simulink model "EHB_speedgoat_R2020a_V1"  (R2020a)
settings: Solver=FixedStepDiscrete  StartTime=0.0  StopTime=inf  FixedStep=0.001  RelTol=1e-3  EnableMultiTasking=on
model workspace (MAT data in the model file):
  A : Simulink.Signal (value not decoded)
  B : Simulink.Signal (value not decoded)
  C : Simulink.Signal (value not decoded)
  D : Simulink.Signal (value not decoded)
  E : Simulink.Signal (value not decoded)
  calin = [-9.96 -7.98 -5.98 -3.99 -1.994 0 1.995 3.992 5.99 7.98 9.97]
  calout = [-10 -8 -6 -4 -2 0 2 4 6 8 10]
symbols that are objects in the model workspace (value not decoded): C, D
undefined symbols (not defined in the file): Com1, none, ts_IO612
libraries: simulink x1436, xpcethercatlib x1223, yisutbxlib_utilities x256, xpcutilitieslib x156, hdlsllib x145, canmsglib x46, speedgoatlib_IO602_4 x11, speedgoatlib_IO611 x7, slrttcplib x4, CanManageLib x3, slrtlib x3, xpcseriallib x2
(part 3 of 30)

== system EHB_speedgoat_R2020a_V1/PowerCtrl/PowerCtrl/CurrSet1 ==
  CurrSet[A] : Inport
  Trigger : TriggerPort  VariantControl=(inherit)  PortDimensions=1
  A2mA : Gain  Gain=1000  OutDataTypeStr=Inherit: Inherit via back propagation
  "Byte Packing " : xpcutilitieslib/Byte Packing   MaskPackedDataType=uint8  MaskUnpackedDataTypes={'uint16'}  MaskAlignment=1
  Byte Packing 1 : xpcutilitieslib/Byte Packing   MaskPackedDataType=uint8  MaskUnpackedDataTypes={'uint16'}  MaskAlignment=1
  CAN Pack : canmsglib/CAN Pack  MsgList=(none)  MsgName=CAN Msg  MsgIDType=Standard (11-bit identifier)  MsgIdentifier=1537  MsgLength=8  Remote=off  ApplyMinMax=off  BusOutput=on  SignalInfo={}
      settings: SourceProductBaseCode=ME,VN  DataFormat=raw data
  CANDataPack_ToUDP : Subsystem
  FunCode : Constant  Value=0x23  OutDataTypeStr=Inherit: Inherit via back propagation
  Index : Constant  Value=0x3003  OutDataTypeStr=Inherit: Inherit via back propagation
  Mux : Mux  Inputs=5
  SubIndex : Constant  Value=0x05  VectorParams1D=off  OutDataTypeStr=Inherit: Inherit via back propagation
  puppet : Constant  Value=[0 0]  OutDataTypeStr=Inherit: Inherit via back propagation
  Output : Outport
  wires:
  CurrSet[A]/1 -> A2mA/1
  puppet/1 -> Mux/5
  SubIndex/1 -> Mux/3
  Index/1 -> "Byte Packing "/1
  A2mA/1 -> Byte Packing 1/1
  Mux/1 -> CAN Pack/1
  "Byte Packing "/1 -> Mux/2
  CAN Pack/1 -> CANDataPack_ToUDP/1(In1)
  Byte Packing 1/1 -> Mux/4
  FunCode/1 -> Mux/1
  CANDataPack_ToUDP/1(Output) -> Output/1

== system EHB_speedgoat_R2020a_V1/PowerCtrl/PowerCtrl/Enable1 ==
  OnOff : Inport
  Trigger : TriggerPort  VariantControl=(inherit)  PortDimensions=1
  "Byte Packing " : xpcutilitieslib/Byte Packing   MaskPackedDataType=uint8  MaskUnpackedDataTypes={'uint16'}  MaskAlignment=1
  CAN Pack1 : canmsglib/CAN Pack  MsgList=(none)  MsgName=CAN Msg  MsgIDType=Standard (11-bit identifier)  MsgIdentifier=1537  MsgLength=8  Remote=off  ApplyMinMax=off  BusOutput=on  SignalInfo={}
      settings: SourceProductBaseCode=ME,VN  DataFormat=raw data
  CANDataPack_ToUDP : Subsystem
  FunCode : Constant  Value=0x2F  OutDataTypeStr=Inherit: Inherit via back propagation
  Index : Constant  Value=0x3002  OutDataTypeStr=Inherit: Inherit via back propagation
  Mux1 : Mux  Inputs=5
  SubIndex : Constant  Value=0x04  VectorParams1D=off  OutDataTypeStr=Inherit: Inherit via back propagation
  puppet : Constant  Value=[0 0 0]  OutDataTypeStr=Inherit: Inherit via back propagation
  Output : Outport
  wires:
  FunCode/1 -> Mux1/1
  puppet/1 -> Mux1/5
  SubIndex/1 -> Mux1/3
  Mux1/1 -> CAN Pack1/1
  CAN Pack1/1 -> CANDataPack_ToUDP/1(In1)
  OnOff/1 -> Mux1/4
  "Byte Packing "/1 -> Mux1/2
  Index/1 -> "Byte Packing "/1
  CANDataPack_ToUDP/1(Output) -> Output/1

== system EHB_speedgoat_R2020a_V1/PowerCtrl/PowerCtrl/IT_M3902D_Ctrl_Trigger ==
  VoltValue : Inport
  OnOff : Inport  Port=2
  CurrSet : Inport  Port=3
  PowerPosSet : Inport  Port=4
  Data Type Conversion : DataTypeConversion
  Data Type Conversion1 : DataTypeConversion
  Data Type Conversion2 : DataTypeConversion  Commented=on
  Detect Change : simulink/Logic and Bit Operations/Detect Change  vinit=0  OutDataTypeStr=boolean
  Mux : Mux  Inputs=5
  Pulse Generator : DiscretePulseGenerator  Commented=on  PulseType=Time based  Period=1  PulseWidth=50
  HVRealy_Ctrl_Trigger : Outport
  wires:
  Detect Change/1 -> HVRealy_Ctrl_Trigger/1  "HVRealy_Ctrl_Trigger"
  Mux/1 -> Detect Change/1
  CurrSet/1 -> Mux/3
  PowerPosSet/1 -> Mux/4
  VoltValue/1 -> Data Type Conversion/1
  OnOff/1 -> Data Type Conversion1/1
  Data Type Conversion/1 -> Mux/1
  Data Type Conversion1/1 -> Mux/2
  Pulse Generator/1 -> Data Type Conversion2/1
  Data Type Conversion2/1 -> Mux/5

== system EHB_speedgoat_R2020a_V1/PowerCtrl/PowerCtrl/PowerPosSet1 ==
  PowerPosSet[W] : Inport
  Trigger : TriggerPort  VariantControl=(inherit)  PortDimensions=1
  "Byte Packing " : xpcutilitieslib/Byte Packing   MaskPackedDataType=uint8  MaskUnpackedDataTypes={'uint16'}  MaskAlignment=1
  Byte Packing 1 : xpcutilitieslib/Byte Packing   MaskPackedDataType=uint8  MaskUnpackedDataTypes={'uint16'}  MaskAlignment=1
  CAN Pack : canmsglib/CAN Pack  MsgList=(none)  MsgName=CAN Msg  MsgIDType=Standard (11-bit identifier)  MsgIdentifier=1537  MsgLength=8  Remote=off  ApplyMinMax=off  BusOutput=on  SignalInfo={}
      settings: SourceProductBaseCode=ME,VN  DataFormat=raw data
  CANDataPack_ToUDP : Subsystem
  FunCode : Constant  Value=0x23  OutDataTypeStr=Inherit: Inherit via back propagation
  Index : Constant  Value=0x3003  OutDataTypeStr=Inherit: Inherit via back propagation
  Mux : Mux  Inputs=5
  SubIndex : Constant  Value=0x0E  VectorParams1D=off  OutDataTypeStr=Inherit: Inherit via back propagation
  W2mW : Gain  Gain=1000  OutDataTypeStr=Inherit: Inherit via back propagation
  puppet : Constant  Value=[0 0]  OutDataTypeStr=Inherit: Inherit via back propagation
  Output : Outport
  wires:
  PowerPosSet[W]/1 -> W2mW/1
  puppet/1 -> Mux/5
  SubIndex/1 -> Mux/3
  Index/1 -> "Byte Packing "/1
  Mux/1 -> CAN Pack/1
  "Byte Packing "/1 -> Mux/2
  CAN Pack/1 -> CANDataPack_ToUDP/1(In1)
  W2mW/1 -> Byte Packing 1/1
  FunCode/1 -> Mux/1
  Byte Packing 1/1 -> Mux/4
  CANDataPack_ToUDP/1(Output) -> Output/1

== system EHB_speedgoat_R2020a_V1/PowerCtrl/PowerCtrl/VoltSet1 ==
  VoltValue[V] : Inport
  Trigger : TriggerPort  VariantControl=(inherit)  PortDimensions=1
  "Byte Packing " : xpcutilitieslib/Byte Packing   MaskPackedDataType=uint8  MaskUnpackedDataTypes={'uint16'}  MaskAlignment=1
  Byte Packing 1 : xpcutilitieslib/Byte Packing   MaskPackedDataType=uint8  MaskUnpackedDataTypes={'uint32'}  MaskAlignment=1
  CAN Pack : canmsglib/CAN Pack  MsgList=(none)  MsgName=CAN Msg  MsgIDType=Standard (11-bit identifier)  MsgIdentifier=1537  MsgLength=8  Remote=off  ApplyMinMax=off  BusOutput=on  SignalInfo={}
      settings: SourceProductBaseCode=ME,VN  DataFormat=raw data
  CANDataPack_ToUDP : Subsystem
  FunCode : Constant  Value=0x23  OutDataTypeStr=Inherit: Inherit via back propagation
  Index : Constant  Value=0x3003  OutDataTypeStr=Inherit: Inherit via back propagation
  Mux : Mux
  SubIndex : Constant  Value=0x02  VectorParams1D=off  OutDataTypeStr=Inherit: Inherit via back propagation
  V2mV : Gain  Gain=1000  OutDataTypeStr=Inherit: Inherit via back propagation
  Output : Outport
  wires:
  FunCode/1 -> Mux/1
  Byte Packing 1/1 -> Mux/4
  CAN Pack/1 -> CANDataPack_ToUDP/1(In1)
  "Byte Packing "/1 -> Mux/2
  Mux/1 -> CAN Pack/1
  V2mV/1 -> Byte Packing 1/1
  Index/1 -> "Byte Packing "/1
  SubIndex/1 -> Mux/3
  VoltValue[V]/1 -> V2mV/1
  CANDataPack_ToUDP/1(Output) -> Output/1

== system EHB_speedgoat_R2020a_V1/TIF_04/CB2020_1/ADC ==
  DTCB CH1 : DataTypeConversion  OutDataTypeStr=double
  DTCB CH2 : DataTypeConversion  OutDataTypeStr=double
  DTCB CH3 : DataTypeConversion  OutDataTypeStr=double
  EtherCAT PDO Receive ADC CH1 : xpcethercatlib/EtherCAT PDO Receive  Priority=2  sig_name=Box 5 (CB2020).PDOGetValue process data mapping.adcvalue1  sig_offset=10808  sig_type=uint16  type_size=16  sig_dim=1  device_id=0  sample_time=0.001000
      settings: SourceProductBaseCode=XP
  EtherCAT PDO Receive ADC CH2 : xpcethercatlib/EtherCAT PDO Receive  Priority=2  sig_name=Box 5 (CB2020).PDOGetValue process data mapping.adcvalue2  sig_offset=10824  sig_type=uint16  type_size=16  sig_dim=1  device_id=0  sample_time=0.001000
      settings: SourceProductBaseCode=XP
  EtherCAT PDO Receive ADC CH3 : xpcethercatlib/EtherCAT PDO Receive  Priority=2  sig_name=Box 5 (CB2020).PDOGetValue process data mapping.adcvalue3  sig_offset=10840  sig_type=uint16  type_size=16  sig_dim=1  device_id=0  sample_time=0.001000
      settings: SourceProductBaseCode=XP
  Gain CH1 : Gain  Gain=1/1000
  Gain CH2 : Gain  Gain=1/1000
  Gain CH3 : Gain  Gain=1/1000
  ADC_CH1[V] : Outport
  ADC_CH2[V] : Outport  Port=2
  ADC_CH3[V] : Outport  Port=3
  wires:
  EtherCAT PDO Receive ADC CH1/1 -> DTCB CH1/1
  DTCB CH1/1 -> Gain CH1/1
  Gain CH1/1 -> ADC_CH1[V]/1  "ADC_CH1[V]"
  EtherCAT PDO Receive ADC CH2/1 -> DTCB CH2/1
  DTCB CH2/1 -> Gain CH2/1
  Gain CH2/1 -> ADC_CH2[V]/1  "ADC_CH2[V]"
  EtherCAT PDO Receive ADC CH3/1 -> DTCB CH3/1
  DTCB CH3/1 -> Gain CH3/1
  Gain CH3/1 -> ADC_CH3[V]/1  "ADC_CH3[V]"

== system EHB_speedgoat_R2020a_V1/TIF_04/CB2020_1/AI1 ==
  Vol : Inport
  Add : Sum  Inputs=-+
  Constant : Constant  Value=4.9874
  V2A : Gain  Gain=1/0.1  OutDataTypeStr=Inherit: Inherit via back propagation
  Cur : Outport
  wires:
  Add/1 -> V2A/1
  Vol/1 -> Add/2
  Constant/1 -> Add/1
  V2A/1 -> Cur/1

== system EHB_speedgoat_R2020a_V1/TIF_04/CB2020_1/AI2 ==
  Vol : Inport
  Add : Sum  Inputs=-+
  Constant : Constant  Value=5.0067
  V2A : Gain  Gain=1/0.1  OutDataTypeStr=Inherit: Inherit via back propagation
  Cur : Outport
  wires:
  V2A/1 -> Cur/1
  Constant/1 -> Add/1
  Vol/1 -> Add/2
  Add/1 -> V2A/1

== system EHB_speedgoat_R2020a_V1/TIF_04/CB2020_1/AI3 ==
  Vol : Inport
  Add : Sum  Inputs=-+
  Constant : Constant  Value=4.9975
  V2A : Gain  Gain=1/0.1  OutDataTypeStr=Inherit: Inherit via back propagation
  Cur : Outport
  wires:
  Add/1 -> V2A/1
  Vol/1 -> Add/2
  Constant/1 -> Add/1
  V2A/1 -> Cur/1

== system EHB_speedgoat_R2020a_V1/TIF_04/CB2020_1/DAC1 ==
  DAC_CH1[V] : Inport
  DAC_CH1_CAL[V] : Constant  Value=0
  EtherCAT PDO Transmit DAC CH1 : xpcethercatlib/EtherCAT PDO Transmit   Priority=3  sig_name=Box 5 (CB2020).PDOSetValue process data mapping.dacvalue1  sig_offset=10808  sig_type=int16  type_size=16  sig_dim=1  device_id=0  sample_time=0.001000
      settings: SourceProductBaseCode=XP
  dp2c CH1 : Subsystem  mask(dacphy2cmd){}
  wires:
  DAC_CH1[V]/1 -> dp2c CH1/1(dac_value)
  DAC_CH1_CAL[V]/1 -> dp2c CH1/2(dac_value_calibrate)
  dp2c CH1/1(cmd_value) -> EtherCAT PDO Transmit DAC CH1/1

== system EHB_speedgoat_R2020a_V1/TIF_04/CB2020_1/mean1 ==
  In1 : Inport
  Add : Sum  Inputs=++++
  Add{1..4} (4 alike) : Sum  Inputs=++++++++++++++++++++
  Delay{,1..79} (80 alike) : Delay  DelayLength=1
  Gain : Gain  Gain=1/80
  Vol : Outport
  wires:
  Add/1 -> Gain/1
  Gain/1 -> Vol/1
  Delay36/1 -> Delay37/1, Add2/7
  Delay37/1 -> Delay38/1, Add2/8
  Delay34/1 -> Delay35/1, Add2/5
  Delay33/1 -> Delay34/1, Add2/4
  Delay20/1 -> Delay21/1, Add2/1
  Delay32/1 -> Delay33/1, Add2/3
  Add2/1 -> Add/2
  Delay35/1 -> Delay36/1, Add2/6
  Delay21/1 -> Delay32/1, Add2/2
  Delay38/1 -> Delay39/1, Add2/9
  Delay39/1 -> Delay22/1, Add2/10
  Delay19/1 -> Add1/20, Delay20/1
  Delay30/1 -> Delay31/1, Add2/19
  Delay23/1 -> Delay24/1, Add2/12
  Delay27/1 -> Delay28/1, Add2/16
  Delay24/1 -> Delay25/1, Add2/13
  Delay22/1 -> Delay23/1, Add2/11
  Delay25/1 -> Delay26/1, Add2/14
  Delay26/1 -> Delay27/1, Add2/15
  Delay29/1 -> Delay30/1, Add2/18
  Delay28/1 -> Delay29/1, Add2/17
  Delay16/1 -> Add1/17, Delay17/1
  Delay17/1 -> Add1/18, Delay18/1
  Delay14/1 -> Add1/15, Delay15/1
  Delay13/1 -> Add1/14, Delay14/1
  Delay10/1 -> Add1/11, Delay11/1
  Delay12/1 -> Add1/13, Delay13/1
  Delay15/1 -> Add1/16, Delay16/1
  Delay11/1 -> Add1/12, Delay12/1
  Delay18/1 -> Add1/19, Delay19/1
  In1/1 -> Delay/1
  Delay9/1 -> Add1/10, Delay10/1
  Delay8/1 -> Add1/9, Delay9/1
  Delay1/1 -> Add1/2, Delay2/1
  Delay5/1 -> Add1/6, Delay6/1
  Add1/1 -> Add/1
  Delay2/1 -> Add1/3, Delay3/1
  Delay/1 -> Add1/1, Delay1/1
  Delay3/1 -> Add1/4, Delay4/1
  Delay4/1 -> Add1/5, Delay5/1
  Delay7/1 -> Add1/8, Delay8/1
  Delay6/1 -> Add1/7, Delay7/1
  Delay48/1 -> Add3/17, Delay49/1
  Delay49/1 -> Add3/18, Delay50/1
  Delay46/1 -> Add3/15, Delay47/1
  Delay45/1 -> Add3/14, Delay46/1
  Delay42/1 -> Add3/11, Delay43/1
  Delay44/1 -> Add3/13, Delay45/1
  Delay47/1 -> Add3/16, Delay48/1
  Delay43/1 -> Add3/12, Delay44/1
  Delay50/1 -> Add3/19, Delay51/1
  Delay31/1 -> Delay40/1, Add2/20
  Delay59/1 -> Add3/10, Delay42/1
  Delay58/1 -> Add3/9, Delay59/1
  Delay41/1 -> Add3/2, Delay52/1
  Delay55/1 -> Add3/6, Delay56/1
  Add3/1 -> Add/3
  Delay52/1 -> Add3/3, Delay53/1
  Delay40/1 -> Add3/1, Delay41/1
  Delay53/1 -> Add3/4, Delay54/1
  Delay54/1 -> Add3/5, Delay55/1
  Delay57/1 -> Add3/8, Delay58/1
  Delay56/1 -> Add3/7, Delay57/1
  Delay76/1 -> Delay77/1, Add4/7
  Delay77/1 -> Delay78/1, Add4/8
  Delay74/1 -> Delay75/1, Add4/5
  Delay73/1 -> Delay74/1, Add4/4
  Delay60/1 -> Delay61/1, Add4/1
  Delay72/1 -> Delay73/1, Add4/3
  Add4/1 -> Add/4
  Delay75/1 -> Delay76/1, Add4/6
  Delay61/1 -> Delay72/1, Add4/2
  Delay78/1 -> Delay79/1, Add4/9
  Delay79/1 -> Delay62/1, Add4/10
  Delay71/1 -> Add4/20
  Delay51/1 -> Delay60/1, Add3/20
  Delay70/1 -> Delay71/1, Add4/19
  Delay63/1 -> Delay64/1, Add4/12
  Delay67/1 -> Delay68/1, Add4/16
  Delay64/1 -> Delay65/1, Add4/13
  Delay62/1 -> Delay63/1, Add4/11
  Delay65/1 -> Delay66/1, Add4/14
  Delay66/1 -> Delay67/1, Add4/15
  Delay69/1 -> Delay70/1, Add4/18
  Delay68/1 -> Delay69/1, Add4/17

== system EHB_speedgoat_R2020a_V1/TIF_04/CB2020_1/mean2 ==
  In1 : Inport
  Add : Sum  Inputs=++++
  Add{1..4} (4 alike) : Sum  Inputs=++++++++++++++++++++
  Delay{,1..79} (80 alike) : Delay  DelayLength=1
  Gain : Gain  Gain=1/80
  Vol : Outport
  wires:
  Delay68/1 -> Add4/17, Delay69/1
  Delay69/1 -> Add4/18, Delay70/1
  Delay66/1 -> Add4/15, Delay67/1
  Delay65/1 -> Add4/14, Delay66/1
  Delay62/1 -> Add4/11, Delay63/1
  Delay64/1 -> Add4/13, Delay65/1
  Delay67/1 -> Add4/16, Delay68/1
  Delay63/1 -> Add4/12, Delay64/1
  Delay70/1 -> Add4/19, Delay71/1
  Delay51/1 -> Add3/20, Delay60/1
  Delay71/1 -> Add4/20
  Delay79/1 -> Add4/10, Delay62/1
  Delay78/1 -> Add4/9, Delay79/1
  Delay61/1 -> Add4/2, Delay72/1
  Delay75/1 -> Add4/6, Delay76/1
  Add4/1 -> Add/4
  Delay72/1 -> Add4/3, Delay73/1
  Delay60/1 -> Add4/1, Delay61/1
  Delay73/1 -> Add4/4, Delay74/1
  Delay74/1 -> Add4/5, Delay75/1
  Delay77/1 -> Add4/8, Delay78/1
  Delay76/1 -> Add4/7, Delay77/1
  Delay56/1 -> Delay57/1, Add3/7
  Delay57/1 -> Delay58/1, Add3/8
  Delay54/1 -> Delay55/1, Add3/5
  Delay53/1 -> Delay54/1, Add3/4
  Delay40/1 -> Delay41/1, Add3/1
  Delay52/1 -> Delay53/1, Add3/3
  Add3/1 -> Add/3
  Delay55/1 -> Delay56/1, Add3/6
  Delay41/1 -> Delay52/1, Add3/2
  Delay58/1 -> Delay59/1, Add3/9
  Delay59/1 -> Delay42/1, Add3/10
  Delay31/1 -> Add2/20, Delay40/1
  Delay50/1 -> Delay51/1, Add3/19
  Delay43/1 -> Delay44/1, Add3/12
  Delay47/1 -> Delay48/1, Add3/16
  Delay44/1 -> Delay45/1, Add3/13
  Delay42/1 -> Delay43/1, Add3/11
  Delay45/1 -> Delay46/1, Add3/14
  Delay46/1 -> Delay47/1, Add3/15
  Delay49/1 -> Delay50/1, Add3/18
  Delay48/1 -> Delay49/1, Add3/17
  Delay6/1 -> Delay7/1, Add1/7
  Delay7/1 -> Delay8/1, Add1/8
  Delay4/1 -> Delay5/1, Add1/5
  Delay3/1 -> Delay4/1, Add1/4
  Delay/1 -> Delay1/1, Add1/1
  Delay2/1 -> Delay3/1, Add1/3
  Add1/1 -> Add/1
  Delay5/1 -> Delay6/1, Add1/6
  Delay1/1 -> Delay2/1, Add1/2
  Delay8/1 -> Delay9/1, Add1/9
  Delay9/1 -> Delay10/1, Add1/10
  In1/1 -> Delay/1
  Delay18/1 -> Delay19/1, Add1/19
  Delay11/1 -> Delay12/1, Add1/12
  Delay15/1 -> Delay16/1, Add1/16
  Delay12/1 -> Delay13/1, Add1/13
  Delay10/1 -> Delay11/1, Add1/11
  Delay13/1 -> Delay14/1, Add1/14
  Delay14/1 -> Delay15/1, Add1/15
  Delay17/1 -> Delay18/1, Add1/18
  Delay16/1 -> Delay17/1, Add1/17
  Delay28/1 -> Add2/17, Delay29/1
  Delay29/1 -> Add2/18, Delay30/1
  Delay26/1 -> Add2/15, Delay27/1
  Delay25/1 -> Add2/14, Delay26/1
  Delay22/1 -> Add2/11, Delay23/1
  Delay24/1 -> Add2/13, Delay25/1
  Delay27/1 -> Add2/16, Delay28/1
  Delay23/1 -> Add2/12, Delay24/1
  Delay30/1 -> Add2/19, Delay31/1
  Delay19/1 -> Delay20/1, Add1/20
  Delay39/1 -> Add2/10, Delay22/1
  Delay38/1 -> Add2/9, Delay39/1
  Delay21/1 -> Add2/2, Delay32/1
  Delay35/1 -> Add2/6, Delay36/1
  Add2/1 -> Add/2
  Delay32/1 -> Add2/3, Delay33/1
  Delay20/1 -> Add2/1, Delay21/1
  Delay33/1 -> Add2/4, Delay34/1
  Delay34/1 -> Add2/5, Delay35/1
  Delay37/1 -> Add2/8, Delay38/1
  Delay36/1 -> Add2/7, Delay37/1
  Gain/1 -> Vol/1
  Add/1 -> Gain/1

== system EHB_speedgoat_R2020a_V1/TIF_04/CB2020_1/mean3 ==
  In1 : Inport
  Add : Sum  Inputs=++++
  Add{1..4} (4 alike) : Sum  Inputs=++++++++++++++++++++
  Delay{,1..79} (80 alike) : Delay  DelayLength=1
  Gain : Gain  Gain=1/80
  Vol : Outport
  wires:
  Add/1 -> Gain/1
  Gain/1 -> Vol/1
  Delay36/1 -> Delay37/1, Add2/7
  Delay37/1 -> Delay38/1, Add2/8
  Delay34/1 -> Delay35/1, Add2/5
  Delay33/1 -> Delay34/1, Add2/4
  Delay20/1 -> Delay21/1, Add2/1
  Delay32/1 -> Delay33/1, Add2/3
  Add2/1 -> Add/2
  Delay35/1 -> Delay36/1, Add2/6
  Delay21/1 -> Delay32/1, Add2/2
  Delay38/1 -> Delay39/1, Add2/9
  Delay39/1 -> Delay22/1, Add2/10
  Delay19/1 -> Add1/20, Delay20/1
  Delay30/1 -> Delay31/1, Add2/19
  Delay23/1 -> Delay24/1, Add2/12
  Delay27/1 -> Delay28/1, Add2/16
  Delay24/1 -> Delay25/1, Add2/13
  Delay22/1 -> Delay23/1, Add2/11
  Delay25/1 -> Delay26/1, Add2/14
  Delay26/1 -> Delay27/1, Add2/15
  Delay29/1 -> Delay30/1, Add2/18
  Delay28/1 -> Delay29/1, Add2/17
  Delay16/1 -> Add1/17, Delay17/1
  Delay17/1 -> Add1/18, Delay18/1
  Delay14/1 -> Add1/15, Delay15/1
  Delay13/1 -> Add1/14, Delay14/1
  Delay10/1 -> Add1/11, Delay11/1
  Delay12/1 -> Add1/13, Delay13/1
  Delay15/1 -> Add1/16, Delay16/1
  Delay11/1 -> Add1/12, Delay12/1
  Delay18/1 -> Add1/19, Delay19/1
  In1/1 -> Delay/1
  Delay9/1 -> Add1/10, Delay10/1
  Delay8/1 -> Add1/9, Delay9/1
  Delay1/1 -> Add1/2, Delay2/1
  Delay5/1 -> Add1/6, Delay6/1
  Add1/1 -> Add/1
  Delay2/1 -> Add1/3, Delay3/1
  Delay/1 -> Add1/1, Delay1/1
  Delay3/1 -> Add1/4, Delay4/1
  Delay4/1 -> Add1/5, Delay5/1
  Delay7/1 -> Add1/8, Delay8/1
  Delay6/1 -> Add1/7, Delay7/1
  Delay48/1 -> Add3/17, Delay49/1
  Delay49/1 -> Add3/18, Delay50/1
  Delay46/1 -> Add3/15, Delay47/1
  Delay45/1 -> Add3/14, Delay46/1
  Delay42/1 -> Add3/11, Delay43/1
  Delay44/1 -> Add3/13, Delay45/1
  Delay47/1 -> Add3/16, Delay48/1
  Delay43/1 -> Add3/12, Delay44/1
  Delay50/1 -> Add3/19, Delay51/1
  Delay31/1 -> Delay40/1, Add2/20
  Delay59/1 -> Add3/10, Delay42/1
  Delay58/1 -> Add3/9, Delay59/1
  Delay41/1 -> Add3/2, Delay52/1
  Delay55/1 -> Add3/6, Delay56/1
  Add3/1 -> Add/3
  Delay52/1 -> Add3/3, Delay53/1
  Delay40/1 -> Add3/1, Delay41/1
  Delay53/1 -> Add3/4, Delay54/1
  Delay54/1 -> Add3/5, Delay55/1
  Delay57/1 -> Add3/8, Delay58/1
  Delay56/1 -> Add3/7, Delay57/1
  Delay76/1 -> Delay77/1, Add4/7
  Delay77/1 -> Delay78/1, Add4/8
  Delay74/1 -> Delay75/1, Add4/5
  Delay73/1 -> Delay74/1, Add4/4
  Delay60/1 -> Delay61/1, Add4/1
  Delay72/1 -> Delay73/1, Add4/3
  Add4/1 -> Add/4
  Delay75/1 -> Delay76/1, Add4/6
  Delay61/1 -> Delay72/1, Add4/2
  Delay78/1 -> Delay79/1, Add4/9
  Delay79/1 -> Delay62/1, Add4/10
  Delay71/1 -> Add4/20
  Delay51/1 -> Delay60/1, Add3/20
  Delay70/1 -> Delay71/1, Add4/19
  Delay63/1 -> Delay64/1, Add4/12
  Delay67/1 -> Delay68/1, Add4/16
  Delay64/1 -> Delay65/1, Add4/13
  Delay62/1 -> Delay63/1, Add4/11
  Delay65/1 -> Delay66/1, Add4/14
  Delay66/1 -> Delay67/1, Add4/15
  Delay69/1 -> Delay70/1, Add4/18
  Delay68/1 -> Delay69/1, Add4/17

== system EHB_speedgoat_R2020a_V1/TIF_04/CB2020_2/ADC ==
  DTCB CH{1..16} (16 alike) : DataTypeConversion  OutDataTypeStr=double
  EtherCAT PDO Receive ADC CH1 : xpcethercatlib/EtherCAT PDO Receive  Priority=2  sig_name=Box 6 (CB2020).PDOGetValue process data mapping.adcvalue1  sig_offset=11128  sig_type=uint16  type_size=16  sig_dim=1  device_id=0  sample_time=0.001000
      settings: SourceProductBaseCode=XP
  EtherCAT PDO Receive ADC CH10 : xpcethercatlib/EtherCAT PDO Receive  Priority=2  sig_name=Box 6 (CB2020).PDOGetValue process data mapping.adcvalue10  sig_offset=11272  sig_type=uint16  type_size=16  sig_dim=1  device_id=0  sample_time=0.001000
      settings: SourceProductBaseCode=XP
  EtherCAT PDO Receive ADC CH11 : xpcethercatlib/EtherCAT PDO Receive  Priority=2  sig_name=Box 6 (CB2020).PDOGetValue process data mapping.adcvalue11  sig_offset=11288  sig_type=uint16  type_size=16  sig_dim=1  device_id=0  sample_time=0.001000
      settings: SourceProductBaseCode=XP
  EtherCAT PDO Receive ADC CH12 : xpcethercatlib/EtherCAT PDO Receive  Priority=2  sig_name=Box 6 (CB2020).PDOGetValue process data mapping.adcvalue12  sig_offset=11304  sig_type=uint16  type_size=16  sig_dim=1  device_id=0  sample_time=0.001000
      settings: SourceProductBaseCode=XP
  EtherCAT PDO Receive ADC CH13 : xpcethercatlib/EtherCAT PDO Receive  Priority=2  sig_name=Box 6 (CB2020).PDOGetValue process data mapping.adcvalue13  sig_offset=11320  sig_type=uint16  type_size=16  sig_dim=1  device_id=0  sample_time=0.001000
      settings: SourceProductBaseCode=XP
  EtherCAT PDO Receive ADC CH14 : xpcethercatlib/EtherCAT PDO Receive  Priority=2  sig_name=Box 6 (CB2020).PDOGetValue process data mapping.adcvalue14  sig_offset=11336  sig_type=uint16  type_size=16  sig_dim=1  device_id=0  sample_time=0.001000
      settings: SourceProductBaseCode=XP
  EtherCAT PDO Receive ADC CH15 : xpcethercatlib/EtherCAT PDO Receive  Priority=2  sig_name=Box 6 (CB2020).PDOGetValue process data mapping.adcvalue15  sig_offset=11352  sig_type=uint16  type_size=16  sig_dim=1  device_id=0  sample_time=0.001000
      settings: SourceProductBaseCode=XP
  EtherCAT PDO Receive ADC CH16 : xpcethercatlib/EtherCAT PDO Receive  Priority=2  sig_name=Box 6 (CB2020).PDOGetValue process data mapping.adcvalue16  sig_offset=11368  sig_type=uint16  type_size=16  sig_dim=1  device_id=0  sample_time=0.001000
      settings: SourceProductBaseCode=XP
  EtherCAT PDO Receive ADC CH2 : xpcethercatlib/EtherCAT PDO Receive  Priority=2  sig_name=Box 6 (CB2020).PDOGetValue process data mapping.adcvalue2  sig_offset=11144  sig_type=uint16  type_size=16  sig_dim=1  device_id=0  sample_time=0.001000
      settings: SourceProductBaseCode=XP
  EtherCAT PDO Receive ADC CH3 : xpcethercatlib/EtherCAT PDO Receive  Priority=2  sig_name=Box 6 (CB2020).PDOGetValue process data mapping.adcvalue3  sig_offset=11160  sig_type=uint16  type_size=16  sig_dim=1  device_id=0  sample_time=0.001000
      settings: SourceProductBaseCode=XP
  EtherCAT PDO Receive ADC CH4 : xpcethercatlib/EtherCAT PDO Receive  Priority=2  sig_name=Box 6 (CB2020).PDOGetValue process data mapping.adcvalue4  sig_offset=11176  sig_type=uint16  type_size=16  sig_dim=1  device_id=0  sample_time=0.001000
      settings: SourceProductBaseCode=XP
  EtherCAT PDO Receive ADC CH5 : xpcethercatlib/EtherCAT PDO Receive  Priority=2  sig_name=Box 6 (CB2020).PDOGetValue process data mapping.adcvalue5  sig_offset=11192  sig_type=uint16  type_size=16  sig_dim=1  device_id=0  sample_time=0.001000
      settings: SourceProductBaseCode=XP
  EtherCAT PDO Receive ADC CH6 : xpcethercatlib/EtherCAT PDO Receive  Priority=2  sig_name=Box 6 (CB2020).PDOGetValue process data mapping.adcvalue6  sig_offset=11208  sig_type=uint16  type_size=16  sig_dim=1  device_id=0  sample_time=0.001000
      settings: SourceProductBaseCode=XP
  EtherCAT PDO Receive ADC CH7 : xpcethercatlib/EtherCAT PDO Receive  Priority=2  sig_name=Box 6 (CB2020).PDOGetValue process data mapping.adcvalue7  sig_offset=11224  sig_type=uint16  type_size=16  sig_dim=1  device_id=0  sample_time=0.001000
      settings: SourceProductBaseCode=XP
  EtherCAT PDO Receive ADC CH8 : xpcethercatlib/EtherCAT PDO Receive  Priority=2  sig_name=Box 6 (CB2020).PDOGetValue process data mapping.adcvalue8  sig_offset=11240  sig_type=uint16  type_size=16  sig_dim=1  device_id=0  sample_time=0.001000
      settings: SourceProductBaseCode=XP
  EtherCAT PDO Receive ADC CH9 : xpcethercatlib/EtherCAT PDO Receive  Priority=2  sig_name=Box 6 (CB2020).PDOGetValue process data mapping.adcvalue9  sig_offset=11256  sig_type=uint16  type_size=16  sig_dim=1  device_id=0  sample_time=0.001000
      settings: SourceProductBaseCode=XP
  Gain CH{1..16} (16 alike) : Gain  Gain=1/1000
  ADC_CH1[V] : Outport
  ADC_CH2[V] : Outport  Port=2
  ADC_CH3[V] : Outport  Port=3
  ADC_CH4[V] : Outport  Port=4
  ADC_CH5[V] : Outport  Port=5
  ADC_CH6[V] : Outport  Port=6
  ADC_CH7[V] : Outport  Port=7
  ADC_CH8[V] : Outport  Port=8
  ADC_CH9[V] : Outport  Port=9
  ADC_CH10[V] : Outport  Port=10
  ADC_CH11[V] : Outport  Port=11
  ADC_CH12[V] : Outport  Port=12
  ADC_CH13[V] : Outport  Port=13
  ADC_CH14[V] : Outport  Port=14
  ADC_CH15[V] : Outport  Port=15
  ADC_CH16[V] : Outport  Port=16
  wires:
  EtherCAT PDO Receive ADC CH1/1 -> DTCB CH1/1
  DTCB CH1/1 -> Gain CH1/1
  Gain CH1/1 -> ADC_CH1[V]/1  "ADC_CH1[V]"
  EtherCAT PDO Receive ADC CH2/1 -> DTCB CH2/1
  DTCB CH2/1 -> Gain CH2/1
  Gain CH2/1 -> ADC_CH2[V]/1  "ADC_CH2[V]"
  EtherCAT PDO Receive ADC CH3/1 -> DTCB CH3/1
  DTCB CH3/1 -> Gain CH3/1
  Gain CH3/1 -> ADC_CH3[V]/1  "ADC_CH3[V]"
  EtherCAT PDO Receive ADC CH4/1 -> DTCB CH4/1
  DTCB CH4/1 -> Gain CH4/1
  Gain CH4/1 -> ADC_CH4[V]/1  "ADC_CH4[V]"
  EtherCAT PDO Receive ADC CH5/1 -> DTCB CH5/1
  DTCB CH5/1 -> Gain CH5/1
  Gain CH5/1 -> ADC_CH5[V]/1  "ADC_CH5[V]"
  EtherCAT PDO Receive ADC CH6/1 -> DTCB CH6/1
  DTCB CH6/1 -> Gain CH6/1
  Gain CH6/1 -> ADC_CH6[V]/1  "ADC_CH6[V]"
  EtherCAT PDO Receive ADC CH7/1 -> DTCB CH7/1
  DTCB CH7/1 -> Gain CH7/1
  Gain CH7/1 -> ADC_CH7[V]/1  "ADC_CH7[V]"
  EtherCAT PDO Receive ADC CH8/1 -> DTCB CH8/1
  DTCB CH8/1 -> Gain CH8/1
  Gain CH8/1 -> ADC_CH8[V]/1  "ADC_CH8[V]"
  EtherCAT PDO Receive ADC CH9/1 -> DTCB CH9/1
  DTCB CH9/1 -> Gain CH9/1
  Gain CH9/1 -> ADC_CH9[V]/1  "ADC_CH9[V]"
  EtherCAT PDO Receive ADC CH10/1 -> DTCB CH10/1
  DTCB CH10/1 -> Gain CH10/1
  Gain CH10/1 -> ADC_CH10[V]/1  "ADC_CH10[V]"
  EtherCAT PDO Receive ADC CH11/1 -> DTCB CH11/1
  DTCB CH11/1 -> Gain CH11/1
  Gain CH11/1 -> ADC_CH11[V]/1  "ADC_CH11[V]"
  EtherCAT PDO Receive ADC CH12/1 -> DTCB CH12/1
  DTCB CH12/1 -> Gain CH12/1
  Gain CH12/1 -> ADC_CH12[V]/1  "ADC_CH12[V]"
  EtherCAT PDO Receive ADC CH13/1 -> DTCB CH13/1
  DTCB CH13/1 -> Gain CH13/1
  Gain CH13/1 -> ADC_CH13[V]/1  "ADC_CH13[V]"
  EtherCAT PDO Receive ADC CH14/1 -> DTCB CH14/1
  DTCB CH14/1 -> Gain CH14/1
  Gain CH14/1 -> ADC_CH14[V]/1  "ADC_CH14[V]"
  EtherCAT PDO Receive ADC CH15/1 -> DTCB CH15/1
  DTCB CH15/1 -> Gain CH15/1
  Gain CH15/1 -> ADC_CH15[V]/1  "ADC_CH15[V]"
  EtherCAT PDO Receive ADC CH16/1 -> DTCB CH16/1
  DTCB CH16/1 -> Gain CH16/1
  Gain CH16/1 -> ADC_CH16[V]/1  "ADC_CH16[V]"

== system EHB_speedgoat_R2020a_V1/TIF_04/CB2020_2/AI1 ==
  Vol : Inport
  Add : Sum  Inputs=-+
  Constant : Constant  Value=4.976
  V2A : Gain  Gain=1/0.1  OutDataTypeStr=Inherit: Inherit via back propagation
  Cur : Outport
  wires:
  Add/1 -> V2A/1
  Vol/1 -> Add/2
  Constant/1 -> Add/1
  V2A/1 -> Cur/1

== system EHB_speedgoat_R2020a_V1/TIF_04/CB2020_2/AI10 ==
  Vol : Inport
  Add : Sum  Inputs=-+
  Constant : Constant  Value=4.9836
  V2A : Gain  Gain=1/0.1  OutDataTypeStr=Inherit: Inherit via back propagation
  Cur : Outport
  wires:
  Add/1 -> V2A/1
  Vol/1 -> Add/2
  Constant/1 -> Add/1
  V2A/1 -> Cur/1

== system EHB_speedgoat_R2020a_V1/TIF_04/CB2020_2/AI11 ==
  Vol : Inport
  Add : Sum  Inputs=-+
  Constant : Constant  Value=5.003
  V2A : Gain  Gain=1/0.1  OutDataTypeStr=Inherit: Inherit via back propagation
  Cur : Outport
  wires:
  V2A/1 -> Cur/1
  Constant/1 -> Add/1
  Vol/1 -> Add/2
  Add/1 -> V2A/1

== system EHB_speedgoat_R2020a_V1/TIF_04/CB2020_2/AI12 ==
  Vol : Inport
  Add : Sum  Inputs=-+
  Constant : Constant  Value=4.994
  V2A : Gain  Gain=1/0.1  OutDataTypeStr=Inherit: Inherit via back propagation
  Cur : Outport
  wires:
  Add/1 -> V2A/1
  Vol/1 -> Add/2
  Constant/1 -> Add/1
  V2A/1 -> Cur/1

== system EHB_speedgoat_R2020a_V1/TIF_04/CB2020_2/AI13 ==
  Vol : Inport
  Add : Sum  Inputs=-+
  Constant : Constant  Value=5
  V2A : Gain  Gain=1/0.1  OutDataTypeStr=Inherit: Inherit via back propagation
  Cur : Outport
  wires:
  V2A/1 -> Cur/1
  Constant/1 -> Add/1
  Vol/1 -> Add/2
  Add/1 -> V2A/1

== system EHB_speedgoat_R2020a_V1/TIF_04/CB2020_2/AI14 ==
  Vol : Inport
  Add : Sum  Inputs=-+
  Constant : Constant  Value=4.996
  V2A : Gain  Gain=1/0.1  OutDataTypeStr=Inherit: Inherit via back propagation
  Cur : Outport
  wires:
  V2A/1 -> Cur/1
  Constant/1 -> Add/1
  Vol/1 -> Add/2
  Add/1 -> V2A/1

== system EHB_speedgoat_R2020a_V1/TIF_04/CB2020_2/AI15 ==
  Vol : Inport
  Add : Sum  Inputs=-+
  Constant : Constant  Value=4.9926
  V2A : Gain  Gain=1/0.1  OutDataTypeStr=Inherit: Inherit via back propagation
  Cur : Outport
  wires:
  Add/1 -> V2A/1
  Vol/1 -> Add/2
  Constant/1 -> Add/1
  V2A/1 -> Cur/1

== system EHB_speedgoat_R2020a_V1/TIF_04/CB2020_2/AI16 ==
  Vol : Inport
  Add : Sum  Inputs=-+
  Constant : Constant  Value=4.996
  V2A : Gain  Gain=1/0.1  OutDataTypeStr=Inherit: Inherit via back propagation
  Cur : Outport
  wires:
  V2A/1 -> Cur/1
  Constant/1 -> Add/1
  Vol/1 -> Add/2
  Add/1 -> V2A/1

== system EHB_speedgoat_R2020a_V1/TIF_04/CB2020_2/AI2 ==
  Vol : Inport
  Add : Sum  Inputs=-+
  Constant : Constant  Value=4.9959
  V2A : Gain  Gain=1/0.1  OutDataTypeStr=Inherit: Inherit via back propagation
  Cur : Outport
  wires:
  V2A/1 -> Cur/1
  Constant/1 -> Add/1
  Vol/1 -> Add/2
  Add/1 -> V2A/1

== system EHB_speedgoat_R2020a_V1/TIF_04/CB2020_2/AI3 ==
  Vol : Inport
  Add : Sum  Inputs=-+
  Constant : Constant  Value=5.0018
  V2A : Gain  Gain=1/0.1  OutDataTypeStr=Inherit: Inherit via back propagation
  Cur : Outport
  wires:
  Add/1 -> V2A/1
  Vol/1 -> Add/2
  Constant/1 -> Add/1
  V2A/1 -> Cur/1

== system EHB_speedgoat_R2020a_V1/TIF_04/CB2020_2/AI4 ==
  Vol : Inport
  Add : Sum  Inputs=-+
  Constant : Constant  Value=5.0032
  V2A : Gain  Gain=1/0.1  OutDataTypeStr=Inherit: Inherit via back propagation
  Cur : Outport
  wires:
  V2A/1 -> Cur/1
  Constant/1 -> Add/1
  Vol/1 -> Add/2
  Add/1 -> V2A/1

== system EHB_speedgoat_R2020a_V1/TIF_04/CB2020_2/AI5 ==
  Vol : Inport
  Add : Sum  Inputs=-+
  Constant : Constant  Value=4.999
  V2A : Gain  Gain=1/0.1  OutDataTypeStr=Inherit: Inherit via back propagation
  Cur : Outport
  wires:
  Add/1 -> V2A/1
  Vol/1 -> Add/2
  Constant/1 -> Add/1
  V2A/1 -> Cur/1

== system EHB_speedgoat_R2020a_V1/TIF_04/CB2020_2/AI6 ==
  Vol : Inport
  Add : Sum  Inputs=-+
  Constant : Constant  Value=4.996
  V2A : Gain  Gain=1/0.1  OutDataTypeStr=Inherit: Inherit via back propagation
  Cur : Outport
  wires:
  V2A/1 -> Cur/1
  Constant/1 -> Add/1
  Vol/1 -> Add/2
  Add/1 -> V2A/1

== system EHB_speedgoat_R2020a_V1/TIF_04/CB2020_2/AI7 ==
  Vol : Inport
  Add : Sum  Inputs=-+
  Constant : Constant  Value=4.9869
  V2A : Gain  Gain=1/0.1  OutDataTypeStr=Inherit: Inherit via back propagation
  Cur : Outport
  wires:
  Add/1 -> V2A/1
  Vol/1 -> Add/2
  Constant/1 -> Add/1
  V2A/1 -> Cur/1

== system EHB_speedgoat_R2020a_V1/TIF_04/CB2020_2/AI8 ==
  Vol : Inport
  Add : Sum  Inputs=-+
  Constant : Constant  Value=4.9817
  V2A : Gain  Gain=1/0.1  OutDataTypeStr=Inherit: Inherit via back propagation
  Cur : Outport
  wires:
  Add/1 -> V2A/1
  Vol/1 -> Add/2
  Constant/1 -> Add/1
  V2A/1 -> Cur/1

== system EHB_speedgoat_R2020a_V1/TIF_04/CB2020_2/AI9 ==
  Vol : Inport
  Add : Sum  Inputs=-+
  Constant : Constant  Value=4.9854
  V2A : Gain  Gain=1/0.1  OutDataTypeStr=Inherit: Inherit via back propagation
  Cur : Outport
  wires:
  V2A/1 -> Cur/1
  Constant/1 -> Add/1
  Vol/1 -> Add/2
  Add/1 -> V2A/1

== system EHB_speedgoat_R2020a_V1/TIF_04/CB2020_2/DAC ==
  DAC_CH1[V] : Inport
  DAC_CH2[V] : Inport  Port=2
  DAC_CH3[V] : Inport  Port=3
  DAC_CH4[V] : Inport  Port=4
  DAC_CH5[V] : Inport  Port=5
  DAC_CH6[V] : Inport  Port=6
  DAC_CH7[V] : Inport  Port=7
  DAC_CH8[V] : Inport  Port=8
  DAC_CH9[V] : Inport  Port=9
  DAC_CH10[V] : Inport  Port=10
  DAC_CH11[V] : Inport  Port=11
  DAC_CH12[V] : Inport  Port=12
  DAC_CH13[V] : Inport  Port=13
  DAC_CH14[V] : Inport  Port=14
  DAC_CH15[V] : Inport  Port=15
  DAC_CH16[V] : Inport  Port=16
  DAC_CH17[V] : Inport  Port=17
  DAC_CH18[V] : Inport  Port=18
  DAC_CH19[V] : Inport  Port=19
  DAC_CH20[V] : Inport  Port=20
  DAC_CH10_CAL[V] : Constant  Value=0
  DAC_CH11_CAL[V] : Constant  Value=0
  DAC_CH12_CAL[V] : Constant  Value=0
  DAC_CH13_CAL[V] : Constant  Value=0
  DAC_CH14_CAL[V] : Constant  Value=0
  DAC_CH15_CAL[V] : Constant  Value=0
  DAC_CH16_CAL[V] : Constant  Value=0
  DAC_CH17_CAL[V] : Constant  Value=0
  DAC_CH18_CAL[V] : Constant  Value=0
  DAC_CH19_CAL[V] : Constant  Value=0
  DAC_CH1_CAL[V] : Constant  Value=0
  DAC_CH20_CAL[V] : Constant  Value=0
  DAC_CH2_CAL[V] : Constant  Value=0
  DAC_CH3_CAL[V] : Constant  Value=0
  DAC_CH4_CAL[V] : Constant  Value=0
  DAC_CH5_CAL[V] : Constant  Value=0
  DAC_CH6_CAL[V] : Constant  Value=0
  DAC_CH7_CAL[V] : Constant  Value=0
  DAC_CH8_CAL[V] : Constant  Value=0
  DAC_CH9_CAL[V] : Constant  Value=0
  EtherCAT PDO Transmit DAC CH1 : xpcethercatlib/EtherCAT PDO Transmit   Priority=3  sig_name=Box 6 (CB2020).PDOSetValue process data mapping.dacvalue1  sig_offset=11128  sig_type=int16  type_size=16  sig_dim=1  device_id=0  sample_time=0.001000
      settings: SourceProductBaseCode=XP
  EtherCAT PDO Transmit DAC CH10 : xpcethercatlib/EtherCAT PDO Transmit   Priority=3  sig_name=Box 6 (CB2020).PDOSetValue process data mapping.dacvalue10  sig_offset=11272  sig_type=int16  type_size=16  sig_dim=1  device_id=0  sample_time=0.001000
      settings: SourceProductBaseCode=XP
  EtherCAT PDO Transmit DAC CH11 : xpcethercatlib/EtherCAT PDO Transmit   Priority=3  sig_name=Box 6 (CB2020).PDOSetValue process data mapping.dacvalue11  sig_offset=11288  sig_type=int16  type_size=16  sig_dim=1  device_id=0  sample_time=0.001000
      settings: SourceProductBaseCode=XP
  EtherCAT PDO Transmit DAC CH12 : xpcethercatlib/EtherCAT PDO Transmit   Priority=3  sig_name=Box 6 (CB2020).PDOSetValue process data mapping.dacvalue12  sig_offset=11304  sig_type=int16  type_size=16  sig_dim=1  device_id=0  sample_time=0.001000
      settings: SourceProductBaseCode=XP
  EtherCAT PDO Transmit DAC CH13 : xpcethercatlib/EtherCAT PDO Transmit   Priority=3  sig_name=Box 6 (CB2020).PDOSetValue process data mapping.dacvalue13  sig_offset=11320  sig_type=int16  type_size=16  sig_dim=1  device_id=0  sample_time=0.001000
      settings: SourceProductBaseCode=XP
  EtherCAT PDO Transmit DAC CH14 : xpcethercatlib/EtherCAT PDO Transmit   Priority=3  sig_name=Box 6 (CB2020).PDOSetValue process data mapping.dacvalue14  sig_offset=11336  sig_type=int16  type_size=16  sig_dim=1  device_id=0  sample_time=0.001000
      settings: SourceProductBaseCode=XP
  EtherCAT PDO Transmit DAC CH15 : xpcethercatlib/EtherCAT PDO Transmit   Priority=3  sig_name=Box 6 (CB2020).PDOSetValue process data mapping.dacvalue15  sig_offset=11352  sig_type=int16  type_size=16  sig_dim=1  device_id=0  sample_time=0.001000
      settings: SourceProductBaseCode=XP
  EtherCAT PDO Transmit DAC CH16 : xpcethercatlib/EtherCAT PDO Transmit   Priority=3  sig_name=Box 6 (CB2020).PDOSetValue process data mapping.dacvalue16  sig_offset=11368  sig_type=int16  type_size=16  sig_dim=1  device_id=0  sample_time=0.001000
      settings: SourceProductBaseCode=XP
  EtherCAT PDO Transmit DAC CH17 : xpcethercatlib/EtherCAT PDO Transmit   Priority=3  sig_name=Box 6 (CB2020).PDOSetValue process data mapping.dacvalue17  sig_offset=11384  sig_type=int16  type_size=16  sig_dim=1  device_id=0  sample_time=0.001000
      settings: SourceProductBaseCode=XP
  EtherCAT PDO Transmit DAC CH18 : xpcethercatlib/EtherCAT PDO Transmit   Priority=3  sig_name=Box 6 (CB2020).PDOSetValue process data mapping.dacvalue18  sig_offset=11400  sig_type=int16  type_size=16  sig_dim=1  device_id=0  sample_time=0.001000
      settings: SourceProductBaseCode=XP
  EtherCAT PDO Transmit DAC CH19 : xpcethercatlib/EtherCAT PDO Transmit   Priority=3  sig_name=Box 6 (CB2020).PDOSetValue process data mapping.dacvalue19  sig_offset=11416  sig_type=int16  type_size=16  sig_dim=1  device_id=0  sample_time=0.001000
      settings: SourceProductBaseCode=XP
  EtherCAT PDO Transmit DAC CH2 : xpcethercatlib/EtherCAT PDO Transmit   Priority=3  sig_name=Box 6 (CB2020).PDOSetValue process data mapping.dacvalue2  sig_offset=11144  sig_type=int16  type_size=16  sig_dim=1  device_id=0  sample_time=0.001000
      settings: SourceProductBaseCode=XP
  EtherCAT PDO Transmit DAC CH20 : xpcethercatlib/EtherCAT PDO Transmit   Priority=3  sig_name=Box 6 (CB2020).PDOSetValue process data mapping.dacvalue20  sig_offset=11432  sig_type=int16  type_size=16  sig_dim=1  device_id=0  sample_time=0.001000
      settings: SourceProductBaseCode=XP
  EtherCAT PDO Transmit DAC CH3 : xpcethercatlib/EtherCAT PDO Transmit   Priority=3  sig_name=Box 6 (CB2020).PDOSetValue process data mapping.dacvalue3  sig_offset=11160  sig_type=int16  type_size=16  sig_dim=1  device_id=0  sample_time=0.001000
      settings: SourceProductBaseCode=XP
  EtherCAT PDO Transmit DAC CH4 : xpcethercatlib/EtherCAT PDO Transmit   Priority=3  sig_name=Box 6 (CB2020).PDOSetValue process data mapping.dacvalue4  sig_offset=11176  sig_type=int16  type_size=16  sig_dim=1  device_id=0  sample_time=0.001000
      settings: SourceProductBaseCode=XP
  EtherCAT PDO Transmit DAC CH5 : xpcethercatlib/EtherCAT PDO Transmit   Priority=3  sig_name=Box 6 (CB2020).PDOSetValue process data mapping.dacvalue5  sig_offset=11192  sig_type=int16  type_size=16  sig_dim=1  device_id=0  sample_time=0.001000
      settings: SourceProductBaseCode=XP
  EtherCAT PDO Transmit DAC CH6 : xpcethercatlib/EtherCAT PDO Transmit   Priority=3  sig_name=Box 6 (CB2020).PDOSetValue process data mapping.dacvalue6  sig_offset=11208  sig_type=int16  type_size=16  sig_dim=1  device_id=0  sample_time=0.001000
      settings: SourceProductBaseCode=XP
  EtherCAT PDO Transmit DAC CH7 : xpcethercatlib/EtherCAT PDO Transmit   Priority=3  sig_name=Box 6 (CB2020).PDOSetValue process data mapping.dacvalue7  sig_offset=11224  sig_type=int16  type_size=16  sig_dim=1  device_id=0  sample_time=0.001000
      settings: SourceProductBaseCode=XP
  EtherCAT PDO Transmit DAC CH8 : xpcethercatlib/EtherCAT PDO Transmit   Priority=3  sig_name=Box 6 (CB2020).PDOSetValue process data mapping.dacvalue8  sig_offset=11240  sig_type=int16  type_size=16  sig_dim=1  device_id=0  sample_time=0.001000
      settings: SourceProductBaseCode=XP
  EtherCAT PDO Transmit DAC CH9 : xpcethercatlib/EtherCAT PDO Transmit   Priority=3  sig_name=Box 6 (CB2020).PDOSetValue process data mapping.dacvalue9  sig_offset=11256  sig_type=int16  type_size=16  sig_dim=1  device_id=0  sample_time=0.001000
      settings: SourceProductBaseCode=XP
  dp2c CH1 : Subsystem  mask(dacphy2cmd){}
  dp2c CH10 : Subsystem  mask(dacphy2cmd){}
  dp2c CH11 : Subsystem  mask(dacphy2cmd){}
  dp2c CH12 : Subsystem  mask(dacphy2cmd){}
  dp2c CH13 : Subsystem  mask(dacphy2cmd){}
  dp2c CH14 : Subsystem  mask(dacphy2cmd){}
  dp2c CH15 : Subsystem  mask(dacphy2cmd){}
  dp2c CH16 : Subsystem  mask(dacphy2cmd){}
  dp2c CH17 : Subsystem  mask(dacphy2cmd){}
  dp2c CH18 : Subsystem  mask(dacphy2cmd){}
  dp2c CH19 : Subsystem  mask(dacphy2cmd){}
  dp2c CH2 : Subsystem  mask(dacphy2cmd){}
  dp2c CH20 : Subsystem  mask(dacphy2cmd){}
  dp2c CH3 : Subsystem  mask(dacphy2cmd){}
  dp2c CH4 : Subsystem  mask(dacphy2cmd){}
  dp2c CH5 : Subsystem  mask(dacphy2cmd){}
  dp2c CH6 : Subsystem  mask(dacphy2cmd){}
  dp2c CH7 : Subsystem  mask(dacphy2cmd){}
  dp2c CH8 : Subsystem  mask(dacphy2cmd){}
  dp2c CH9 : Subsystem  mask(dacphy2cmd){}
  wires:
  DAC_CH1[V]/1 -> dp2c CH1/1(dac_value)
  DAC_CH1_CAL[V]/1 -> dp2c CH1/2(dac_value_calibrate)
  dp2c CH1/1(cmd_value) -> EtherCAT PDO Transmit DAC CH1/1
  DAC_CH2[V]/1 -> dp2c CH2/1(dac_value)
  DAC_CH2_CAL[V]/1 -> dp2c CH2/2(dac_value_calibrate)
  dp2c CH2/1(cmd_value) -> EtherCAT PDO Transmit DAC CH2/1
  DAC_CH3[V]/1 -> dp2c CH3/1(dac_value)
  DAC_CH3_CAL[V]/1 -> dp2c CH3/2(dac_value_calibrate)
  dp2c CH3/1(cmd_value) -> EtherCAT PDO Transmit DAC CH3/1
  DAC_CH4[V]/1 -> dp2c CH4/1(dac_value)
  DAC_CH4_CAL[V]/1 -> dp2c CH4/2(dac_value_calibrate)
  dp2c CH4/1(cmd_value) -> EtherCAT PDO Transmit DAC CH4/1
  DAC_CH5[V]/1 -> dp2c CH5/1(dac_value)
  DAC_CH5_CAL[V]/1 -> dp2c CH5/2(dac_value_calibrate)
  dp2c CH5/1(cmd_value) -> EtherCAT PDO Transmit DAC CH5/1
  DAC_CH6[V]/1 -> dp2c CH6/1(dac_value)
  DAC_CH6_CAL[V]/1 -> dp2c CH6/2(dac_value_calibrate)
  dp2c CH6/1(cmd_value) -> EtherCAT PDO Transmit DAC CH6/1
  DAC_CH7[V]/1 -> dp2c CH7/1(dac_value)
  DAC_CH7_CAL[V]/1 -> dp2c CH7/2(dac_value_calibrate)
  dp2c CH7/1(cmd_value) -> EtherCAT PDO Transmit DAC CH7/1
  DAC_CH8[V]/1 -> dp2c CH8/1(dac_value)
  DAC_CH8_CAL[V]/1 -> dp2c CH8/2(dac_value_calibrate)
  dp2c CH8/1(cmd_value) -> EtherCAT PDO Transmit DAC CH8/1
  DAC_CH9[V]/1 -> dp2c CH9/1(dac_value)
  DAC_CH9_CAL[V]/1 -> dp2c CH9/2(dac_value_calibrate)
  dp2c CH9/1(cmd_value) -> EtherCAT PDO Transmit DAC CH9/1
  DAC_CH10[V]/1 -> dp2c CH10/1(dac_value)
  DAC_CH10_CAL[V]/1 -> dp2c CH10/2(dac_value_calibrate)
  dp2c CH10/1(cmd_value) -> EtherCAT PDO Transmit DAC CH10/1
  DAC_CH11[V]/1 -> dp2c CH11/1(dac_value)
  DAC_CH11_CAL[V]/1 -> dp2c CH11/2(dac_value_calibrate)
  dp2c CH11/1(cmd_value) -> EtherCAT PDO Transmit DAC CH11/1
  DAC_CH12[V]/1 -> dp2c CH12/1(dac_value)
  DAC_CH12_CAL[V]/1 -> dp2c CH12/2(dac_value_calibrate)
  dp2c CH12/1(cmd_value) -> EtherCAT PDO Transmit DAC CH12/1
  DAC_CH13[V]/1 -> dp2c CH13/1(dac_value)
  DAC_CH13_CAL[V]/1 -> dp2c CH13/2(dac_value_calibrate)
  dp2c CH13/1(cmd_value) -> EtherCAT PDO Transmit DAC CH13/1
  DAC_CH14[V]/1 -> dp2c CH14/1(dac_value)
  DAC_CH14_CAL[V]/1 -> dp2c CH14/2(dac_value_calibrate)
  dp2c CH14/1(cmd_value) -> EtherCAT PDO Transmit DAC CH14/1
  DAC_CH15[V]/1 -> dp2c CH15/1(dac_value)
  DAC_CH15_CAL[V]/1 -> dp2c CH15/2(dac_value_calibrate)
  dp2c CH15/1(cmd_value) -> EtherCAT PDO Transmit DAC CH15/1
  DAC_CH16[V]/1 -> dp2c CH16/1(dac_value)
  DAC_CH16_CAL[V]/1 -> dp2c CH16/2(dac_value_calibrate)
  dp2c CH16/1(cmd_value) -> EtherCAT PDO Transmit DAC CH16/1
  DAC_CH17[V]/1 -> dp2c CH17/1(dac_value)
  DAC_CH17_CAL[V]/1 -> dp2c CH17/2(dac_value_calibrate)
  dp2c CH17/1(cmd_value) -> EtherCAT PDO Transmit DAC CH17/1
  DAC_CH18[V]/1 -> dp2c CH18/1(dac_value)
  DAC_CH18_CAL[V]/1 -> dp2c CH18/2(dac_value_calibrate)
  dp2c CH18/1(cmd_value) -> EtherCAT PDO Transmit DAC CH18/1
  DAC_CH19[V]/1 -> dp2c CH19/1(dac_value)
  DAC_CH19_CAL[V]/1 -> dp2c CH19/2(dac_value_calibrate)
  dp2c CH19/1(cmd_value) -> EtherCAT PDO Transmit DAC CH19/1
  DAC_CH20[V]/1 -> dp2c CH20/1(dac_value)
  DAC_CH20_CAL[V]/1 -> dp2c CH20/2(dac_value_calibrate)
  dp2c CH20/1(cmd_value) -> EtherCAT PDO Transmit DAC CH20/1

== system EHB_speedgoat_R2020a_V1/TIF_04/CB2020_2/mean1 ==
  In1 : Inport
  Add : Sum  Inputs=++++
  Add{1..4} (4 alike) : Sum  Inputs=++++++++++++++++++++
  Delay{,1..79} (80 alike) : Delay  DelayLength=1
  Gain : Gain  Gain=1/80
  Vol : Outport
  wires:
  Add/1 -> Gain/1
  Gain/1 -> Vol/1
  Delay36/1 -> Delay37/1, Add2/7
  Delay37/1 -> Delay38/1, Add2/8
  Delay34/1 -> Delay35/1, Add2/5
  Delay33/1 -> Delay34/1, Add2/4
  Delay20/1 -> Delay21/1, Add2/1
  Delay32/1 -> Delay33/1, Add2/3
  Add2/1 -> Add/2
  Delay35/1 -> Delay36/1, Add2/6
  Delay21/1 -> Delay32/1, Add2/2
  Delay38/1 -> Delay39/1, Add2/9
  Delay39/1 -> Delay22/1, Add2/10
  Delay19/1 -> Add1/20, Delay20/1
  Delay30/1 -> Delay31/1, Add2/19
  Delay23/1 -> Delay24/1, Add2/12
  Delay27/1 -> Delay28/1, Add2/16
  Delay24/1 -> Delay25/1, Add2/13
  Delay22/1 -> Delay23/1, Add2/11
  Delay25/1 -> Delay26/1, Add2/14
  Delay26/1 -> Delay27/1, Add2/15
  Delay29/1 -> Delay30/1, Add2/18
  Delay28/1 -> Delay29/1, Add2/17
  Delay16/1 -> Add1/17, Delay17/1
  Delay17/1 -> Add1/18, Delay18/1
  Delay14/1 -> Add1/15, Delay15/1
  Delay13/1 -> Add1/14, Delay14/1
  Delay10/1 -> Add1/11, Delay11/1
  Delay12/1 -> Add1/13, Delay13/1
  Delay15/1 -> Add1/16, Delay16/1
  Delay11/1 -> Add1/12, Delay12/1
  Delay18/1 -> Add1/19, Delay19/1
  In1/1 -> Delay/1
  Delay9/1 -> Add1/10, Delay10/1
  Delay8/1 -> Add1/9, Delay9/1
  Delay1/1 -> Add1/2, Delay2/1
  Delay5/1 -> Add1/6, Delay6/1
  Add1/1 -> Add/1
  Delay2/1 -> Add1/3, Delay3/1
  Delay/1 -> Add1/1, Delay1/1
  Delay3/1 -> Add1/4, Delay4/1
  Delay4/1 -> Add1/5, Delay5/1
  Delay7/1 -> Add1/8, Delay8/1
  Delay6/1 -> Add1/7, Delay7/1
  Delay48/1 -> Add3/17, Delay49/1
  Delay49/1 -> Add3/18, Delay50/1
  Delay46/1 -> Add3/15, Delay47/1
  Delay45/1 -> Add3/14, Delay46/1
  Delay42/1 -> Add3/11, Delay43/1
  Delay44/1 -> Add3/13, Delay45/1
  Delay47/1 -> Add3/16, Delay48/1
  Delay43/1 -> Add3/12, Delay44/1
  Delay50/1 -> Add3/19, Delay51/1
  Delay31/1 -> Delay40/1, Add2/20
  Delay59/1 -> Add3/10, Delay42/1
  Delay58/1 -> Add3/9, Delay59/1
  Delay41/1 -> Add3/2, Delay52/1
  Delay55/1 -> Add3/6, Delay56/1
  Add3/1 -> Add/3
  Delay52/1 -> Add3/3, Delay53/1
  Delay40/1 -> Add3/1, Delay41/1
  Delay53/1 -> Add3/4, Delay54/1
  Delay54/1 -> Add3/5, Delay55/1
  Delay57/1 -> Add3/8, Delay58/1
  Delay56/1 -> Add3/7, Delay57/1
  Delay76/1 -> Delay77/1, Add4/7
  Delay77/1 -> Delay78/1, Add4/8
  Delay74/1 -> Delay75/1, Add4/5
  Delay73/1 -> Delay74/1, Add4/4
  Delay60/1 -> Delay61/1, Add4/1
  Delay72/1 -> Delay73/1, Add4/3
  Add4/1 -> Add/4
  Delay75/1 -> Delay76/1, Add4/6
  Delay61/1 -> Delay72/1, Add4/2
  Delay78/1 -> Delay79/1, Add4/9
  Delay79/1 -> Delay62/1, Add4/10
  Delay71/1 -> Add4/20
  Delay51/1 -> Delay60/1, Add3/20
  Delay70/1 -> Delay71/1, Add4/19
  Delay63/1 -> Delay64/1, Add4/12
  Delay67/1 -> Delay68/1, Add4/16
  Delay64/1 -> Delay65/1, Add4/13
  Delay62/1 -> Delay63/1, Add4/11
  Delay65/1 -> Delay66/1, Add4/14
  Delay66/1 -> Delay67/1, Add4/15
  Delay69/1 -> Delay70/1, Add4/18
  Delay68/1 -> Delay69/1, Add4/17

== system EHB_speedgoat_R2020a_V1/TIF_04/CB2020_2/mean10 ==
  In1 : Inport
  Add : Sum  Inputs=++++
  Add{1..4} (4 alike) : Sum  Inputs=++++++++++++++++++++
  Delay{,1..79} (80 alike) : Delay  DelayLength=1
  Gain : Gain  Gain=1/80
  Vol : Outport
  wires:
  Delay68/1 -> Add4/17, Delay69/1
  Delay69/1 -> Add4/18, Delay70/1
  Delay66/1 -> Add4/15, Delay67/1
  Delay65/1 -> Add4/14, Delay66/1
  Delay62/1 -> Add4/11, Delay63/1
  Delay64/1 -> Add4/13, Delay65/1
  Delay67/1 -> Add4/16, Delay68/1
  Delay63/1 -> Add4/12, Delay64/1
  Delay70/1 -> Add4/19, Delay71/1
  Delay51/1 -> Add3/20, Delay60/1
  Delay71/1 -> Add4/20
  Delay79/1 -> Add4/10, Delay62/1
  Delay78/1 -> Add4/9, Delay79/1
  Delay61/1 -> Add4/2, Delay72/1
  Delay75/1 -> Add4/6, Delay76/1
  Add4/1 -> Add/4
  Delay72/1 -> Add4/3, Delay73/1
  Delay60/1 -> Add4/1, Delay61/1
  Delay73/1 -> Add4/4, Delay74/1
  Delay74/1 -> Add4/5, Delay75/1
  Delay77/1 -> Add4/8, Delay78/1
  Delay76/1 -> Add4/7, Delay77/1
  Delay56/1 -> Delay57/1, Add3/7
  Delay57/1 -> Delay58/1, Add3/8
  Delay54/1 -> Delay55/1, Add3/5
  Delay53/1 -> Delay54/1, Add3/4
  Delay40/1 -> Delay41/1, Add3/1
  Delay52/1 -> Delay53/1, Add3/3
  Add3/1 -> Add/3
  Delay55/1 -> Delay56/1, Add3/6
  Delay41/1 -> Delay52/1, Add3/2
  Delay58/1 -> Delay59/1, Add3/9
  Delay59/1 -> Delay42/1, Add3/10
  Delay31/1 -> Add2/20, Delay40/1
  Delay50/1 -> Delay51/1, Add3/19
  Delay43/1 -> Delay44/1, Add3/12
  Delay47/1 -> Delay48/1, Add3/16
  Delay44/1 -> Delay45/1, Add3/13
  Delay42/1 -> Delay43/1, Add3/11
  Delay45/1 -> Delay46/1, Add3/14
  Delay46/1 -> Delay47/1, Add3/15
  Delay49/1 -> Delay50/1, Add3/18
  Delay48/1 -> Delay49/1, Add3/17
  Delay6/1 -> Delay7/1, Add1/7
  Delay7/1 -> Delay8/1, Add1/8
  Delay4/1 -> Delay5/1, Add1/5
  Delay3/1 -> Delay4/1, Add1/4
  Delay/1 -> Delay1/1, Add1/1
  Delay2/1 -> Delay3/1, Add1/3
  Add1/1 -> Add/1
  Delay5/1 -> Delay6/1, Add1/6
  Delay1/1 -> Delay2/1, Add1/2
  Delay8/1 -> Delay9/1, Add1/9
  Delay9/1 -> Delay10/1, Add1/10
  In1/1 -> Delay/1
  Delay18/1 -> Delay19/1, Add1/19
  Delay11/1 -> Delay12/1, Add1/12
  Delay15/1 -> Delay16/1, Add1/16
  Delay12/1 -> Delay13/1, Add1/13
  Delay10/1 -> Delay11/1, Add1/11
  Delay13/1 -> Delay14/1, Add1/14
  Delay14/1 -> Delay15/1, Add1/15
  Delay17/1 -> Delay18/1, Add1/18
  Delay16/1 -> Delay17/1, Add1/17
  Delay28/1 -> Add2/17, Delay29/1
  Delay29/1 -> Add2/18, Delay30/1
  Delay26/1 -> Add2/15, Delay27/1
  Delay25/1 -> Add2/14, Delay26/1
  Delay22/1 -> Add2/11, Delay23/1
  Delay24/1 -> Add2/13, Delay25/1
  Delay27/1 -> Add2/16, Delay28/1
  Delay23/1 -> Add2/12, Delay24/1
  Delay30/1 -> Add2/19, Delay31/1
  Delay19/1 -> Delay20/1, Add1/20
  Delay39/1 -> Add2/10, Delay22/1
  Delay38/1 -> Add2/9, Delay39/1
  Delay21/1 -> Add2/2, Delay32/1
  Delay35/1 -> Add2/6, Delay36/1
  Add2/1 -> Add/2
  Delay32/1 -> Add2/3, Delay33/1
  Delay20/1 -> Add2/1, Delay21/1
  Delay33/1 -> Add2/4, Delay34/1
  Delay34/1 -> Add2/5, Delay35/1
  Delay37/1 -> Add2/8, Delay38/1
  Delay36/1 -> Add2/7, Delay37/1
  Gain/1 -> Vol/1
  Add/1 -> Gain/1
